simulink model "Problem18_model"  (R2020b)
settings: Solver=ode4  StartTime=0.0  StopTime=SIM_TIME  FixedStep=STEP_SIZE  RelTol=1e-3
values from neighbouring files (symbols this model uses):
  a4 = 0.98    [Problem7_9.m]    (also in calc_h.m; problem13.m; problem15.m; problem16.m)
  d1 = 1.5    [calc_h.m]    (also in problem17.m; problem18.m; problem20.m; problem21.m)
  F = [tf([f1(1),f2(1)],1) ... (first row only)    [problem12.m]    (also in problem13.m; problem15.m = [tf([f2(1), f1(1), f0],1); problem17.m = [tf([f2(1), f1(1), f0],1); problem18.m = [tf([f2(1), f1(1), f0],1))
  FP = [tf(1,[fp2(1), fp1(1), fp0]) ... (first row only)    [problem17.m]    (also in problem18.m)
  G = 1/n^2 ./ Jeff    [problem13.m]    (also in problem15.m = tf([1/n^2, 0],1); problem17.m = tf([1/n^2, 0],1); problem18.m = tf([1/n^2, 0],1))
  N = [tf([n3(1), n2(1), n1(1), n0],1) ... (first row only)    [problem15.m]    (also in problem17.m; problem18.m)
  T_L = h    [problem13.m]    (also in problem15.m = zeros(4,1); problem16.m = zeros(4,1); problem17.m = abs(h); problem18.m = abs(h))
libraries: cstblocks x12
settings Model: Creator=Theis  LastModifiedBy=Theis

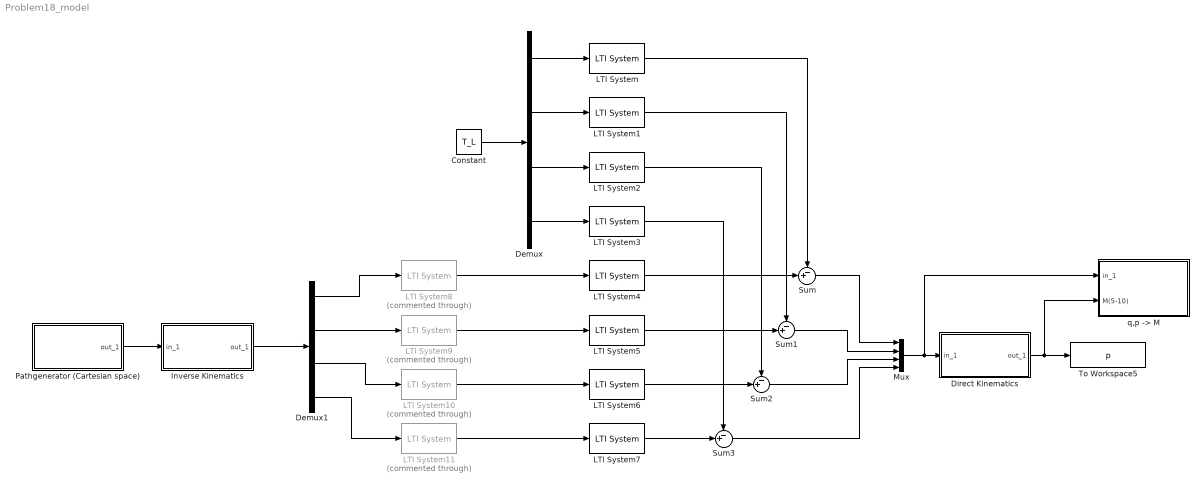
== system Problem18_model ==
  Constant : Constant  Value=T_L
  Demux : Demux
  Demux1 : Demux
  Direct Kinematics : Subsystem
      mask Display: disp('Alto-Robot')
  Inverse Kinematics : Subsystem
      mask Display: disp('Alto-Robot')
  LTI System : cstblocks/LTI System  sys=G/N(1)  IC=[]
  LTI System1 : cstblocks/LTI System  sys=G/N(2)  IC=[]
  LTI System10 : cstblocks/LTI System  Commented=through  sys=FP(3)  IC=[]
  LTI System11 : cstblocks/LTI System  Commented=through  sys=FP(4)  IC=[]
  LTI System2 : cstblocks/LTI System  sys=G/N(3)  IC=[]
  LTI System3 : cstblocks/LTI System  sys=G/N(4)  IC=[]
  LTI System4 : cstblocks/LTI System  sys=F(1)/N(1)  IC=[]
  LTI System5 : cstblocks/LTI System  sys=F(2)/N(2)  IC=[]
  LTI System6 : cstblocks/LTI System  sys=F(3)/N(3)  IC=[]
  LTI System7 : cstblocks/LTI System  sys=F(4)/N(4)  IC=[]
  LTI System8 : cstblocks/LTI System  Commented=through  sys=FP(1)  IC=[]
  LTI System9 : cstblocks/LTI System  Commented=through  sys=FP(2)  IC=[]
  Mux : Mux
  "Pathgenerator (Cartesian space) " : Subsystem
      mask Display: disp('Alto-Robot\nPath -> p')
  Sum{,1..3} (4 alike) : Sum  Inputs=-+|
  To Workspace5 : ToWorkspace  VariableName=p  SaveFormat=Timeseries  SampleTime=-1
  "q,p -> M" : Subsystem
      mask Display: disp('Save to vis4link')
  wires:
  Mux/1 -> Direct Kinematics/1(in_1), "q,p -> M"/1(in_1)
  Sum/1 -> Mux/1
  Sum1/1 -> Mux/2
  Sum2/1 -> Mux/3
  Sum3/1 -> Mux/4
  LTI System10/1 -> LTI System6/1
  LTI System9/1 -> LTI System5/1
  LTI System8/1 -> LTI System4/1
  LTI System11/1 -> LTI System7/1
  Constant/1 -> Demux/1
  LTI System4/1 -> Sum/2
  LTI System5/1 -> Sum1/2
  LTI System6/1 -> Sum2/2
  LTI System7/1 -> Sum3/2
  Demux/1 -> LTI System/1
  Demux/2 -> LTI System1/1
  Demux/3 -> LTI System2/1
  Demux/4 -> LTI System3/1
  LTI System3/1 -> Sum3/1
  LTI System2/1 -> Sum2/1
  LTI System1/1 -> Sum1/1
  LTI System/1 -> Sum/1
  Demux1/4 -> LTI System11/1
  Demux1/3 -> LTI System10/1
  Demux1/2 -> LTI System9/1
  Demux1/1 -> LTI System8/1
  Inverse Kinematics/1(out_1) -> Demux1/1
  Direct Kinematics/1(out_1) -> "q,p -> M"/2(M(5-10)), To Workspace5/1
  "Pathgenerator (Cartesian space) "/1(out_1) -> Inverse Kinematics/1(in_1)

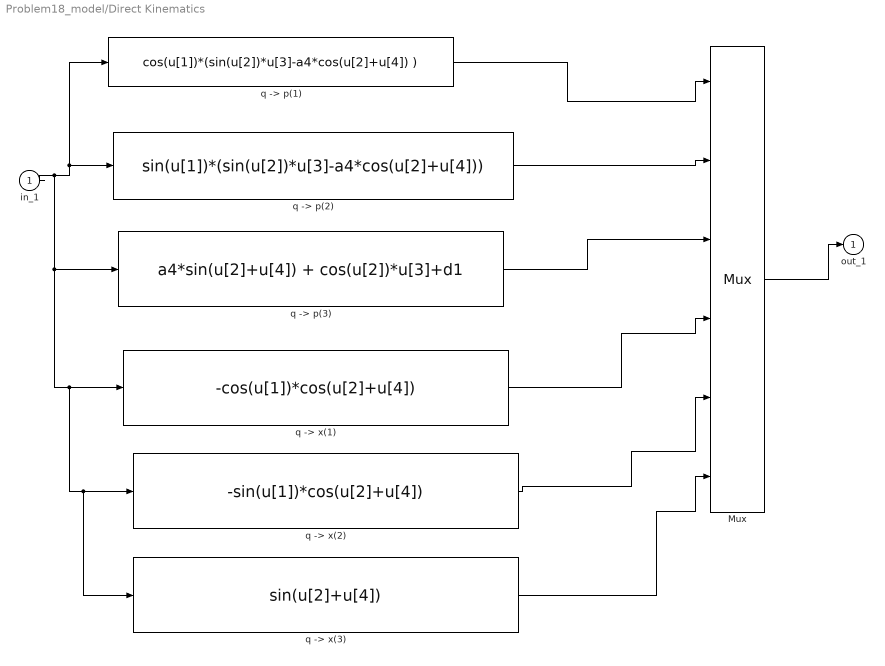
== system Problem18_model/Direct Kinematics ==
  in_1 : Inport
  Mux : Mux  Inputs=6
  "q -> p(1)" : Fcn  Expr=cos(u[1])*(sin(u[2])*u[3]-a4*cos(u[2]+u[4]) )
  "q -> p(2)" : Fcn  Expr=sin(u[1])*(sin(u[2])*u[3]-a4*cos(u[2]+u[4]))
  "q -> p(3)" : Fcn  Expr=a4*sin(u[2]+u[4]) + cos(u[2])*u[3]+d1
  "q -> x(1)" : Fcn  Expr=-cos(u[1])*cos(u[2]+u[4])
  "q -> x(2)" : Fcn  Expr=-sin(u[1])*cos(u[2]+u[4])
  "q -> x(3)" : Fcn  Expr=sin(u[2]+u[4])
  out_1 : Outport  InitialOutput=0  VectorParamsAs1DForOutWhenUnconnected=off
  wires:
  Mux/1 -> out_1/1
  in_1/1 -> "q -> x(3)"/1, "q -> x(2)"/1, "q -> x(1)"/1, "q -> p(3)"/1, "q -> p(2)"/1, "q -> p(1)"/1
  "q -> x(3)"/1 -> Mux/6
  "q -> x(2)"/1 -> Mux/5
  "q -> x(1)"/1 -> Mux/4
  "q -> p(1)"/1 -> Mux/1
  "q -> p(2)"/1 -> Mux/2
  "q -> p(3)"/1 -> Mux/3

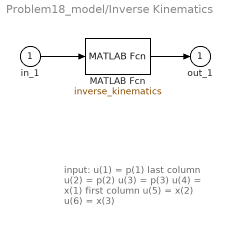
== system Problem18_model/Inverse Kinematics ==
  note: input:
      | u(1) = p(1) last column
      | u(2) = p(2)
      | u(3) = p(3)
      | u(4) = x(1) first column
      | u(5) = x(2)
      | u(6) = x(3)
  in_1 : Inport
  MATLAB Fcn : MATLABFcn  MATLABFcn=inverse_kinematics  OutputDimensions=4
  out_1 : Outport  VectorParamsAs1DForOutWhenUnconnected=off
  wires:
  MATLAB Fcn/1 -> out_1/1
  in_1/1 -> MATLAB Fcn/1

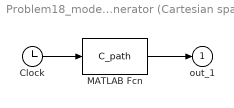
== system Problem18_model/Pathgenerator (Cartesian space)  ==
  Clock : Clock
  MATLAB Fcn : MATLABFcn  MATLABFcn=C_path  OutputDimensions=6
  out_1 : Outport  VectorParamsAs1DForOutWhenUnconnected=off
  wires:
  Clock/1 -> MATLAB Fcn/1
  MATLAB Fcn/1 -> out_1/1

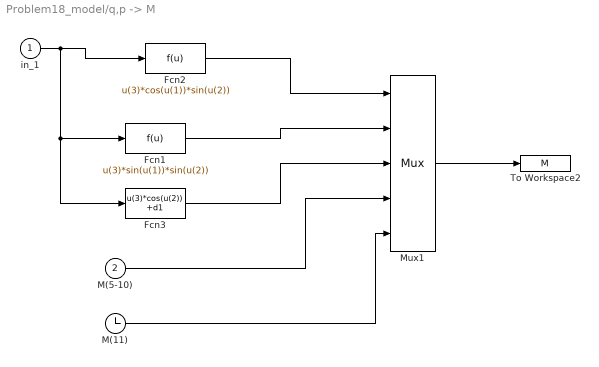
== system Problem18_model/q,p -> M ==
  in_1 : Inport
  M(5-10) : Inport  Port=2
  Fcn1 : Fcn  Expr=u(3)*sin(u(1))*sin(u(2))
  Fcn2 : Fcn  Expr=u(3)*cos(u(1))*sin(u(2))
  Fcn3 : Fcn  Expr=u(3)*cos(u(2)) +d1
  M(11) : Clock
  Mux1 : Mux  Inputs=[1 1 1 6 1]
  To Workspace2 : ToWorkspace  VariableName=M
      settings: MaxDataPoints=100000
  wires:
  M(11)/1 -> Mux1/5
  M(5-10)/1 -> Mux1/4
  Fcn3/1 -> Mux1/3
  Fcn1/1 -> Mux1/2
  Fcn2/1 -> Mux1/1
  in_1/1 -> Fcn3/1, Fcn1/1, Fcn2/1
  Mux1/1 -> To Workspace2/1
